simulink model "Eg5_11"  (R2018a)
settings: Solver=VariableStepAuto  StartTime=0.0  StopTime=10.0  RelTol=1e-3
settings Model: Creator=wangluo  LastModifiedBy=wangluo

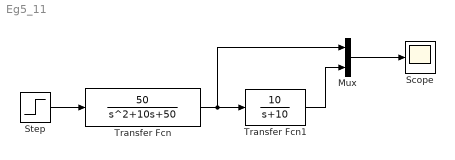
== system Eg5_11 ==
  Mux : Mux  Inputs=2
  Scope : Scope
  Step : Step  SampleTime=0
  Transfer Fcn : TransferFcn  Numerator=[50]  Denominator=[1 10 50]
  Transfer Fcn1 : TransferFcn  Numerator=[10]  Denominator=[1 10]
  wires:
  Step/1 -> Transfer Fcn/1
  Transfer Fcn/1 -> Mux/1, Transfer Fcn1/1
  Mux/1 -> Scope/1
  Transfer Fcn1/1 -> Mux/2
